simulink model "codeee_2_"  (R2026a)
settings: Solver=VariableStepAuto  StopTime=0.2
settings Model: Creator=Mandisa Dlamini  LastModifiedBy=Mandisa Dlamini

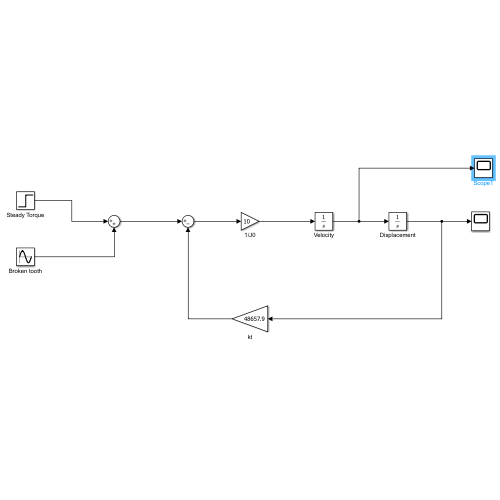
[thumbnail: Simulink's stored preview of the top-level diagram]
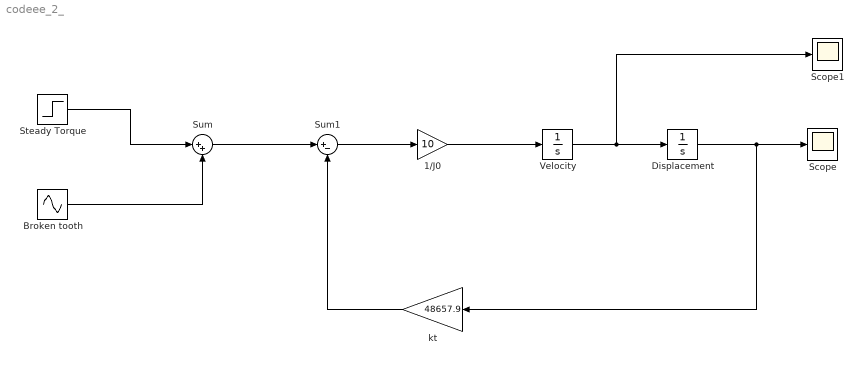
== system codeee_2_ ==
  1/J0 : Gain  Gain=10
  Broken tooth : Sin  Amplitude=200  Frequency=1675.54  SampleTime=0
  Displacement : Integrator
  Scope : Scope
      settings: ActiveDisplayYMinimum=-0.0062076565926088515  ActiveDisplayYMaximum=0.047328087688256144
  Scope1 : Scope
      settings: ActiveDisplayYMinimum=-0.0062076565926088515  ActiveDisplayYMaximum=0.047328087688256144
  Steady Torque : Step  Time=0  FinalValue=1000  SampleTime=0
  Sum : Sum  Inputs=|++
  Sum1 : Sum  Inputs=|+-
  Velocity : Integrator
  kt : Gain  Gain=48657.9
  wires:
  Broken tooth/1 -> Sum/2
  Steady Torque/1 -> Sum/1
  Sum/1 -> Sum1/1
  Sum1/1 -> 1/J0/1
  1/J0/1 -> Velocity/1
  Velocity/1 -> Scope1/1, Displacement/1
  kt/1 -> Sum1/2
  Displacement/1 -> kt/1, Scope/1
